simulink model "DK_FlatnessBased_Template0x2810x293"  (R2024a)
settings: Solver=ode3  StartTime=0.0  StopTime=inf  FixedStep=1e-3  RelTol=1e-5  EnableMultiTasking=on
PostLoadFcn:
  | , if any(exist('dsrtsu_mdlpostloadfcn', 'file') == [2, 3, 6]), try dsrtsu_mdlpostloadfcn('Execute', bdroot); catch fprintf('Error in PostLoadFcn (dsrtsu_mdlpostloadfcn) for model "%s":\n %s\n', bdroot, lasterr); end, end,
InitFcn:
  | k3 = -2;
  | k2 = 3;
  | k1 = 0;
  | k0 = 0;
  | 
  | Kp1 = 0.1;
  | Ki1 = 1;
  | Kp2 = 0.01;
  | Ki2 = 0.1;
  | T = 1;
  | delta_t=0.005;
  | 
  | phi_d=.5;
  | phi_0=0;
  | 
  | Phi_LHP = 0;
  | R = 2.0;
  | Cm = 4.19*exp(-3);
  | L = 20*exp(-6);
  | J = 1.7*exp(-6);
  | Cf = 2.2*exp(-4);
  | D = 1*exp(-7);
  | Mfr = 1*exp(-6);
  | Mpre = 1*exp(-6);
  | 
  | %p0=730000;
  | %p1=23300;
  | p0 = 550000;
  | p1 = 21500;
  | p2=260;
  | 
  | % BesselPole Polynom 4. Ordnung
  | bessel_poles_4 = [-0.6573+0.8302i  ,      -0.6573-0.8302i   ,      -0.9047+0.2711i   ,   -0.9047-0.2711i ]
  | a = poly(bessel_poles_4*15);
undefined symbols (not defined in the file): Ki, Kp, phi, ts
libraries: rtilib1104 x4
settings Model: DSRTSU_INTERNAL_RTI_VER=460  DSRTSU_INTERNAL_RTI_TYPE=rti1104  DSRTSU_INTERNAL_RTIFPGA=50  Creator=7eus  LastModifiedBy=danie
settings SolverCC: AlgebraicLoopSolver=TrustRegion
settings DataIOCC: LimitDataPoints=on  SaveFormat=Array  SignalLoggingSaveFormat=ModelDataLogs  ReturnWorkspaceOutputs=off
settings OptimizationCC: BlockReduction=off  OptimizeBlockIOStorage=off  BufferReuse=off  GlobalBufferReuse=off  ExpressionFolding=off  ExpressionDepthLimit=2147483647  LocalBlockOutputs=off  LifeSpan=inf
settings DebuggingCC: AlgebraicLoopMsg=none  UnderspecifiedInitializationDetection=Classic  MergeDetectMultiDrivingBlocksExec=none  FcnCallInpInsideContextMsg=warning  UnconnectedInputMsg=warning  UnconnectedOutputMsg=warning  UnconnectedLineMsg=warning  StateNameClashWarn=warning  SFUnexpectedBacktrackingDiag=warning  SFNoUnconditionalDefaultTransitionDiag=warning  SFExecutionAtInitializationDiag=none  ArithmeticOperatorsInVariantConditions=warning
settings HardwareCC: ProdBitPerPointer=32  ProdBitPerSizeT=32  ProdBitPerPtrDiffT=32  ProdLargestAtomicFloat=None  ProdEndianess=BigEndian  ProdWordSize=32  ProdHWDeviceType=Generic->Custom  TargetIntDivRoundTo=Zero  TargetEndianess=BigEndian  TargetHWDeviceType=Generic->Custom
settings ModelReferenceCC: EnableRefExpFcnMdlSchedulingChecks=on  PropagateSignalLabelsOutOfModel=off
settings SFSimCC: SimUseLocalCustomCode=off  CustomCodeUndefinedFunction=UseInterfaceOnly
settings RTWCC: Description=dSPACE DS1104 Hardware Platform  SystemTargetFile=rti1104.tlc  MakeCommand=make_rti  TemplateMakefile=rti1104.tmf  RTWUseLocalCustomCode=off  GPUComputeCapability=3.5  DLArmComputeVersion=19.05
settings CodeAppCC: StateflowObjectComments=on
settings STFCustomTargetCC: TargetLangStandard=C89/C90 (ANSI)  ParMdlRefBuildCompliant=on  UseToolchainInfoCompliant=off  SystemTargetFile=rti1104.tlc
settings GRTTargetCC: TargetLangStandard=C89/C90 (ANSI)  CompOptLevelCompliant=off  ConcurrentExecutionCompliant=off  CombineOutputUpdateFcns=off  MatFileLogging=off  CPPClassGenCompliant=off  GRTInterface=on  UseToolchainInfoCompliant=off  ExtModeMexFile=noextcomm
settings ConfigComp: CovMetricSettings=dw  CovSaveCumulativeToWorkspaceVar=on  CovSaveSingleToWorkspaceVar=on  CovExternalEMLEnable=off

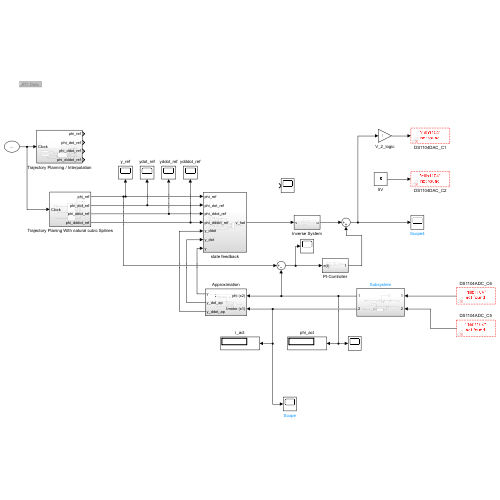
[thumbnail: Simulink's stored preview of the top-level diagram]
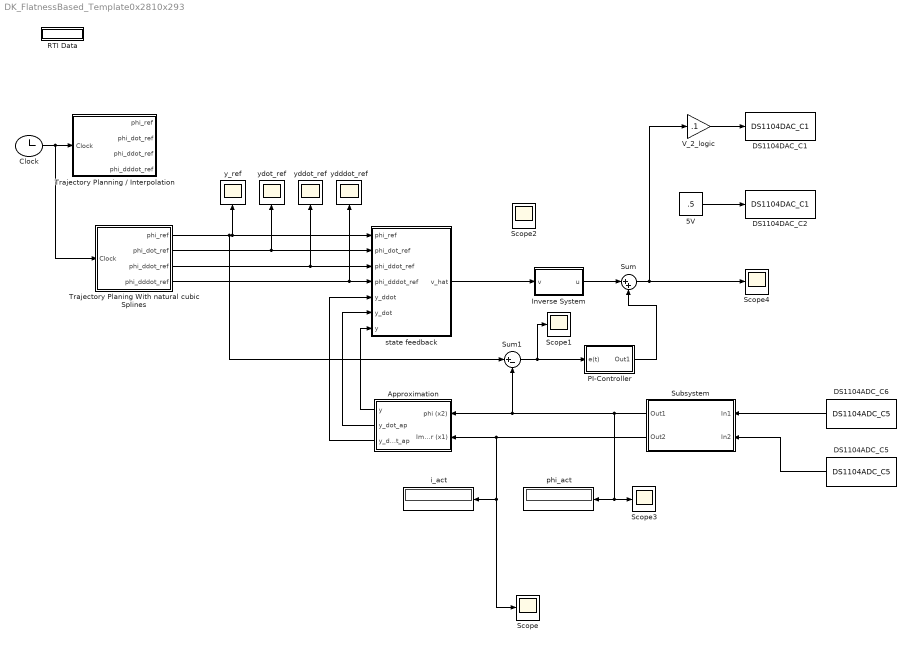
== system DK_FlatnessBased_Template0x2810x293 ==
  5V : Constant  Value=.5
  Approximation : Subsystem
  Clock : Clock
  DS1104ADC_C5 : rtilib1104/DS1104 MASTER PPC/DS1104ADC_C5  ChannelNo=5  TriggerMode=0  Reserved1=[]  Reserved2=[]  Reserved3=[]  Reserved4=[]  DialogFcn=gui1104adc  UnitName={ 'DS1104ADC_C' }  UnitValues={ 5 }  DSProperties=struct('RTI',struct('Version',uint32(1),'BlockType',struct('isSLSource',uint8(1),'isSLSink',uint8(0),'isHWSource',uint8(1),'isHWSink',uint8(0),'isSetup',uint8(0),'isInline',uint8(1),'isNonInline',uint8(0),'isInterrupt',uint8(0),'isChannelwise',uint8(1)),'IOBoardType','DS1104MASTER','UnitType','ADC','Identifier','ADC','DialogType','ML','BlockSet','NONE','SlaveProcessor','NONE'))
  DS1104ADC_C6 : rtilib1104/DS1104 MASTER PPC/DS1104ADC_C5  ChannelNo=6  TriggerMode=0  Reserved1=[]  Reserved2=[]  Reserved3=[]  Reserved4=[]  DialogFcn=gui1104adc  UnitName={ 'DS1104ADC_C' }  UnitValues={6}  DSProperties=struct('RTI',struct('Version',uint32(1),'BlockType',struct('isSLSource',uint8(1),'isSLSink',uint8(0),'isHWSource',uint8(1),'isHWSink',uint8(0),'isSetup',uint8(0),'isInline',uint8(1),'isNonInline',uint8(0),'isInterrupt',uint8(0),'isChannelwise',uint8(1)),'IOBoardType','DS1104MASTER','UnitType','ADC','Identifier','ADC','DialogType','ML','BlockSet','NONE','SlaveProcessor','NONE'))
  DS1104DAC_C1 : rtilib1104/DS1104 MASTER PPC/DS1104DAC_C1  ChannelNo=1  InitValue=0  TermMode=0  TermValue=0  Reserved1=[]  Reserved2=[]  Reserved3=[]  Reserved4=[]  DialogFcn=gui1104dac  UnitName={ 'DS1104DAC_C'}  UnitValues={ 1 }  DSProperties=struct('RTI',struct('Version',uint32(1),'BlockType',struct('isSLSource',uint8(0),'isSLSink',uint8(1),'isHWSource',uint8(0),'isHWSink',uint8(1),'isSetup',uint8(0),'isInline',uint8(1),'isNonInline',uint8(0),'isInterrupt',uint8(0),'isChannelwise',uint8(1)),'IOBoardType','DS1104MASTER','UnitType','DAC','Identifier','DAC','DialogType','ML','BlockSet','NONE','SlaveProcessor','NONE'))
  DS1104DAC_C2 : rtilib1104/DS1104 MASTER PPC/DS1104DAC_C1  ChannelNo=2  InitValue=0  TermMode=0  TermValue=0  Reserved1=[]  Reserved2=[]  Reserved3=[]  Reserved4=[]  DialogFcn=gui1104dac  UnitName={ 'DS1104DAC_C'}  UnitValues={2}  DSProperties=struct('RTI',struct('Version',uint32(1),'BlockType',struct('isSLSource',uint8(0),'isSLSink',uint8(1),'isHWSource',uint8(0),'isHWSink',uint8(1),'isSetup',uint8(0),'isInline',uint8(1),'isNonInline',uint8(0),'isInterrupt',uint8(0),'isChannelwise',uint8(1)),'IOBoardType','DS1104MASTER','UnitType','DAC','Identifier','DAC','DialogType','ML','BlockSet','NONE','SlaveProcessor','NONE'))
  Inverse System : Subsystem
  PI-Controller : Subsystem
  RTI Data : Subsystem  Tag=struct('RTIDataServer',struct('RTIDataServerVs','2','RTIModelDescription','struct(''main'',''DK_FlatnessBased_Template'',''sub'',''DK_FlatnessBased_Template'',''isMp'',0)'))  LoadFcn="if exist('rtidc'), try,  rtidc('DataHostBlockClbLoad', gcbh); catch, disp(['Warning: ''LoadFcn'' for RTI Data block failed: ' lasterr]); end, end,"  mask(RTI_DATA_HOST){}
      mask help:
      | RTI Data Block.
      | This block is used by RTI to store internal model-dependent data.
      | Please keep this block on the root level of the model. Deleting this block will result in data loss.
      |
      | NEVER DELETE OR COPY THIS BLOCK!
      settings: CopyFcn="if exist('rtidc'), try,  rtidc('DataHostBlockClbCopy', gcbh); catch, disp(['Warning: ''CopyFcn'' for RTI Data block failed: ' lasterr]); end, end,"  DeleteFcn="if exist('rtidc'), try,  rtidc('DataHostBlockClbDelete', gcbh); catch, disp(['Warning: ''DeleteFcn'' for RTI Data block failed: ' lasterr]); end, end,"  ModelCloseFcn="if exist('rtidc'), try,  rtidc('DataHostBlockClbModelClose', gcbh); catch, disp(['Warning: ''ModelCloseFcn'' for RTI Data block failed: ' lasterr]); end, end,"  PreSaveFcn="if exist('rtidc'), try,  rtidc('DataHostBlockClbPreSave', gcbh); catch, disp(['Warning: ''PreSaveFcn'' for RTI Data block failed: ' lasterr]); end, end,"  PostSaveFcn="if exist('rtidc'), try,  rtidc('DataHostBlockClbPostSave', gcbh); catch, disp(['Warning: ''PostSaveFcn'' for RTI Data block failed: ' lasterr]); end, end,"  NameChangeFcn="if exist('rtidc'), try,  rtidc('DataHostBlockClbNameChange', gcbh); catch, disp(['Warning: ''NameChangeFcn'' for RTI Data block failed: ' lasterr]); end, end,"
      mask Help:
      | RTI Data Block.
      | This block is used by RTI to store internal model-dependent data.
      | Please keep this block on the root level of the model. Deleting this block will result in data loss.
      | 
      | NEVER DELETE OR COPY THIS BLOCK!
      mask Display: text(0.5, 0.5, 'RTI Data', 'HorizontalAlignment', 'center');
  Scope{,1..4} (5 alike) : Scope
  Subsystem : Subsystem
  Sum : Sum  Inputs=|++
  Sum1 : Sum  Inputs=|+-
  Trajectory Planing With natural cubic Splines : Subsystem
  Trajectory Planning / Interpolation : Subsystem
  V_2_logic : Gain  Gain=.1
  i_act : Display
  phi_act : Display
  state feedback : Subsystem
  y_ref : Scope
  ydddot_ref : Scope
  yddot_ref : Scope
  ydot_ref : Scope
  wires:
  5V/1 -> DS1104DAC_C2/1
  V_2_logic/1 -> DS1104DAC_C1/1
  Trajectory Planing With natural cubic Splines/1(phi_ref) -> y_ref/1, state feedback/1(phi_ref), Sum1/1
  Trajectory Planing With natural cubic Splines/4(phi_dddot_ref) -> ydddot_ref/1, state feedback/4(phi_dddot_ref)
  Approximation/3(y_ddot_ap) -> state feedback/5(y_ddot)
  Approximation/2(y_dot_ap) -> state feedback/6(y_dot)
  Clock/1 -> Trajectory Planing With natural cubic Splines/1(Clock), Trajectory Planning / Interpolation/1(Clock)
  Trajectory Planing With natural cubic Splines/2(phi_dot_ref) -> ydot_ref/1, state feedback/2(phi_dot_ref)
  Approximation/1(y) -> state feedback/7(y)
  Trajectory Planing With natural cubic Splines/3(phi_ddot_ref) -> yddot_ref/1, state feedback/3(phi_ddot_ref)
  state feedback/1(v_hat) -> Inverse System/1(v)
  PI-Controller/1(Out1) -> Sum/2
  Inverse System/1(u) -> Sum/1
  Sum/1 -> Scope4/1, V_2_logic/1
  Sum1/1 -> PI-Controller/1(e(t)), Scope1/1
  Subsystem/1(Out1) -> Sum1/2, Approximation/1(phi (x2)), Scope3/1, phi_act/1
  Subsystem/2(Out2) -> Scope/1, i_act/1, Approximation/2(Imotor (x1))
  DS1104ADC_C6/1 -> Subsystem/1(In1)
  DS1104ADC_C5/1 -> Subsystem/2(In2)

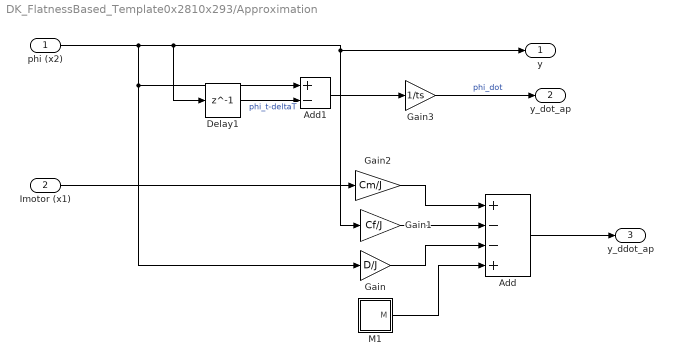
== system DK_FlatnessBased_Template0x2810x293/Approximation ==
  phi (x2) : Inport
  Imotor (x1) : Inport  Port=2
  Add : Sum  Inputs=+--+
  Add1 : Sum  Inputs=+-
  Delay1 : Delay  DelayLength=1  SampleTime=ts
  Gain : Gain  Gain=D/J
  Gain1 : Gain  Gain=Cf/J
  Gain2 : Gain  Gain=Cm/J
  Gain3 : Gain  Gain=1/ts
  M1 : Subsystem
  y : Outport
  y_dot_ap : Outport  Port=2
  y_ddot_ap : Outport  Port=3
  wires:
  phi (x2)/1 -> Gain/1, Add1/1, Delay1/1, Gain1/1, y/1
  M1/1(M) -> Add/4
  Gain/1 -> Add/3
  Gain1/1 -> Add/2
  Gain2/1 -> Add/1
  Imotor (x1)/1 -> Gain2/1
  Add/1 -> y_ddot_ap/1
  Gain3/1 -> y_dot_ap/1  "phi_dot"
  Add1/1 -> Gain3/1
  Delay1/1 -> Add1/2  "phi_t-deltaT"

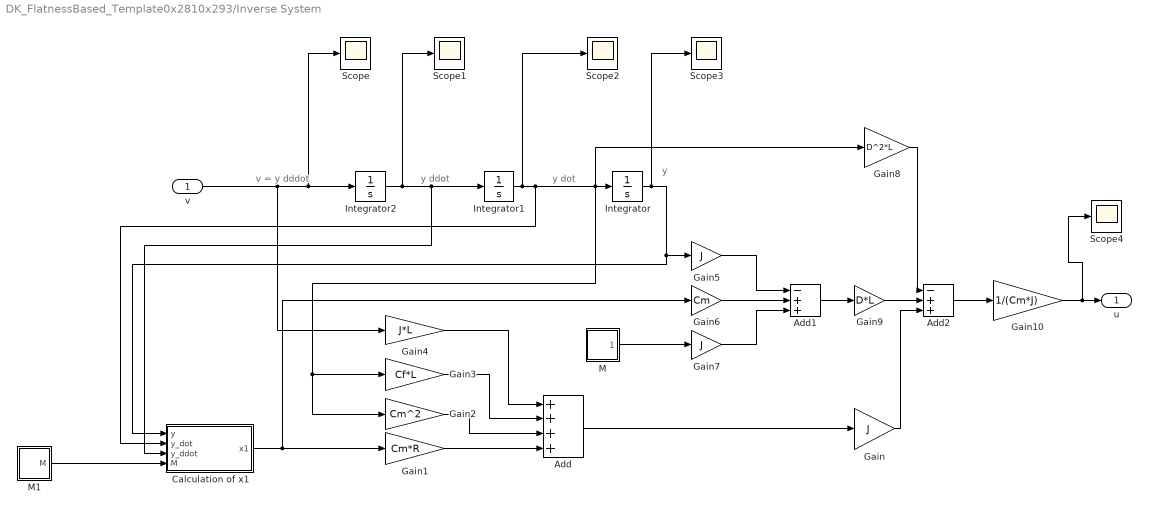
== system DK_FlatnessBased_Template0x2810x293/Inverse System ==
  note: v = y dddot
  note: y ddot
  note: y dot
  note: y
  v : Inport
  Add : Sum  Inputs=++++
  Add1 : Sum  Inputs=-++
  Add2 : Sum  Inputs=-++
  Calculation of x1 : Subsystem
  Gain : Gain  Gain=J
  Gain1 : Gain  Gain=Cm*R
  Gain10 : Gain  Gain=1/(Cm*J)
  Gain2 : Gain  Gain=Cm^2
  Gain3 : Gain  Gain=Cf*L
  Gain4 : Gain  Gain=J*L
  Gain5 : Gain  Gain=J
  Gain6 : Gain  Gain=Cm
  Gain7 : Gain  Gain=J
  Gain8 : Gain  Gain=D^2*L
  Gain9 : Gain  Gain=D*L
  Integrator : Integrator
  Integrator1 : Integrator
  Integrator2 : Integrator
  M : Subsystem
  M1 : Subsystem
  Scope{,1..4} (5 alike) : Scope
  u : Outport
  wires:
  Integrator1/1 -> Scope2/1, Calculation of x1/2(y_dot), Gain8/1, Gain2/1, Gain3/1, Integrator/1
  Integrator2/1 -> Scope1/1, Calculation of x1/3(y_ddot), Integrator1/1
  Integrator/1 -> Scope3/1, Calculation of x1/1(y), Gain5/1
  v/1 -> Scope/1, Integrator2/1, Gain4/1
  Add/1 -> Gain/1
  Gain1/1 -> Add/4
  Gain2/1 -> Add/3
  Gain3/1 -> Add/2
  Gain4/1 -> Add/1
  M/1(Out1) -> Gain7/1
  Gain7/1 -> Add1/3
  Gain6/1 -> Add1/2
  Gain5/1 -> Add1/1
  Add1/1 -> Gain9/1
  Gain10/1 -> Scope4/1, u/1
  Add2/1 -> Gain10/1
  Gain/1 -> Add2/3
  Gain9/1 -> Add2/2
  Gain8/1 -> Add2/1
  Calculation of x1/1(x1) -> Gain6/1, Gain1/1
  M1/1(M) -> Calculation of x1/4(M)

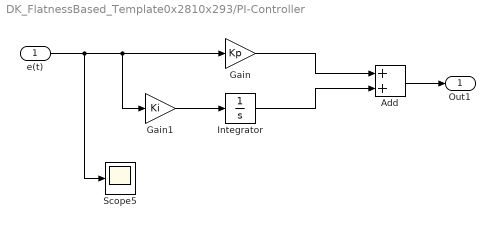
== system DK_FlatnessBased_Template0x2810x293/PI-Controller ==
  e(t) : Inport
  Add : Sum
  Gain : Gain  Gain=Kp
  Gain1 : Gain  Gain=Ki
  Integrator : Integrator
  Scope5 : Scope
  Out1 : Outport
  wires:
  Add/1 -> Out1/1
  e(t)/1 -> Scope5/1, Gain1/1, Gain/1
  Gain/1 -> Add/1
  Integrator/1 -> Add/2
  Gain1/1 -> Integrator/1

== system DK_FlatnessBased_Template0x2810x293/RTI Data ==
  RTI Data Store : Subsystem  mask(RTI_DATA_STORE){}
      mask help:
      | RTI Data Store Block. This block is used by RTI to store internal model dependent data. Deleting this block will result in data loss.
      |
      | NEVER DELETE, COPY, OR MODIFY THIS BLOCK!
      mask Help:
      | RTI Data Store Block. This block is used by RTI to store internal model dependent data. Deleting this block will result in data loss.
      | 
      | NEVER DELETE, COPY, OR MODIFY THIS BLOCK!
      mask Display: text(0.5, 0.5, ' ', 'HorizontalAlignment', 'center');

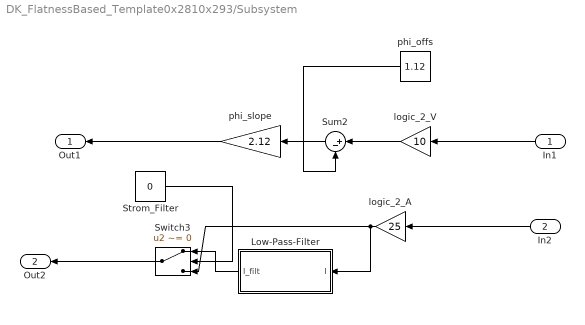
== system DK_FlatnessBased_Template0x2810x293/Subsystem ==
  In1 : Inport
  In2 : Inport  Port=2
  Low-Pass-Filter : Subsystem
  Strom_Filter : Constant  Value=0
  Sum2 : Sum  Inputs=|+-
  Switch3 : Switch  Criteria=u2 ~= 0  SaturateOnIntegerOverflow=off  InputSameDT=off
  logic_2_A : Gain  Gain=25
  logic_2_V : Gain  Gain=10
  phi_offs : Constant  Value=1.12
  phi_slope : Gain  Gain=2.12
  Out1 : Outport
  Out2 : Outport  Port=2
  wires:
  phi_slope/1 -> Out1/1
  Switch3/1 -> Out2/1
  phi_offs/1 -> Sum2/2
  Low-Pass-Filter/1(I_filt) -> Switch3/1
  logic_2_A/1 -> Switch3/3, Low-Pass-Filter/1(I)
  In1/1 -> logic_2_V/1
  Sum2/1 -> phi_slope/1
  logic_2_V/1 -> Sum2/1
  Strom_Filter/1 -> Switch3/2
  In2/1 -> logic_2_A/1

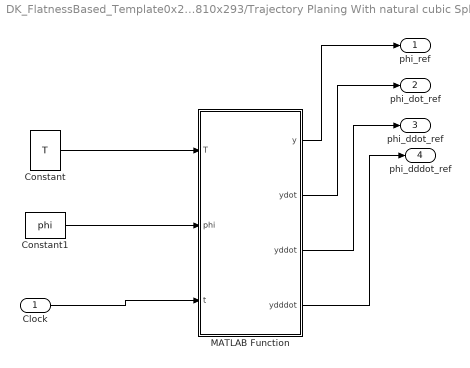
== system DK_FlatnessBased_Template0x2810x293/Trajectory Planing With natural cubic Splines ==
  Clock : Inport
  Constant : Constant  Value=T
  Constant1 : Constant  Value=phi
  MATLAB Function : MATLAB Function  TreatAsAtomicUnit=on
  phi_ref : Outport
  phi_dot_ref : Outport  Port=2
  phi_ddot_ref : Outport  Port=3
  phi_dddot_ref : Outport  Port=4
  wires:
  MATLAB Function/4(ydddot) -> phi_dddot_ref/1
  MATLAB Function/2(ydot) -> phi_dot_ref/1
  MATLAB Function/1(y) -> phi_ref/1
  MATLAB Function/3(yddot) -> phi_ddot_ref/1
  Clock/1 -> MATLAB Function/3(t)
  Constant1/1 -> MATLAB Function/2(phi)
  Constant/1 -> MATLAB Function/1(T)

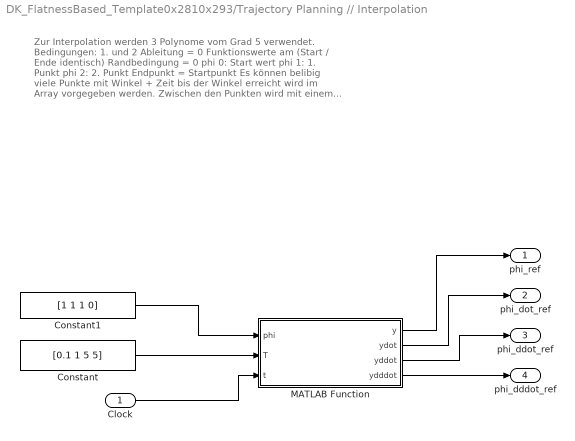
== system DK_FlatnessBased_Template0x2810x293/Trajectory Planning // Interpolation ==
  note: Zur Interpolation werden 3 Polynome vom Grad 5 verwendet.
      |
      | Bedingungen: 1. und 2 Ableitung = 0
      | 			 Funktionswerte am (Start / Ende identisch)
      | 			 Randbedingung = 0
      |
      | phi 0: Start wert
      | phi 1: 1. Punkt
      | phi 2: 2. Punkt
      | Endpunkt = Startpunkt
      |
      | Es können belibig viele Punkte mit Winkel + Zeit bis der Winkel erreicht wird im Array vorgegeben werden.
      |
      | Zwischen den Punkten wird mit einem Polynom 5. Ordnung interpoliert
  Clock : Inport
  Constant : Constant  Value=[0.1 1 5 5]  VectorParams1D=off
  Constant1 : Constant  Value=[1 1 1 0]
  MATLAB Function : MATLAB Function  TreatAsAtomicUnit=on
  phi_ref : Outport
  phi_dot_ref : Outport  Port=2
  phi_ddot_ref : Outport  Port=3
  phi_dddot_ref : Outport  Port=4
  wires:
  MATLAB Function/1(y) -> phi_ref/1
  MATLAB Function/2(ydot) -> phi_dot_ref/1
  MATLAB Function/3(yddot) -> phi_ddot_ref/1
  MATLAB Function/4(ydddot) -> phi_dddot_ref/1
  Clock/1 -> MATLAB Function/3(t)
  Constant/1 -> MATLAB Function/2(T)
  Constant1/1 -> MATLAB Function/1(phi)

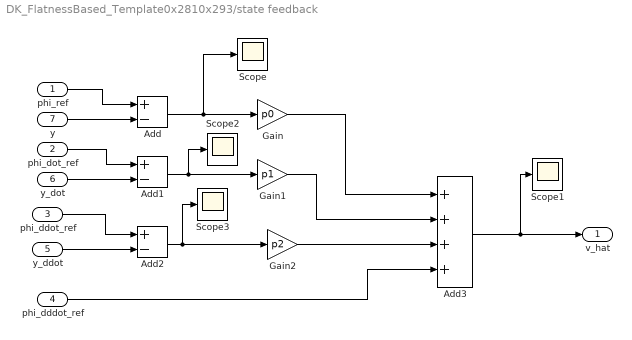
== system DK_FlatnessBased_Template0x2810x293/state feedback ==
  phi_ref : Inport
  phi_dot_ref : Inport  Port=2
  phi_ddot_ref : Inport  Port=3
  phi_dddot_ref : Inport  Port=4
  y_ddot : Inport  Port=5
  y_dot : Inport  Port=6
  y : Inport  Port=7
  Add : Sum  Inputs=+-
  Add1 : Sum  Inputs=+-
  Add2 : Sum  Inputs=+-
  Add3 : Sum  Inputs=++++
  Gain : Gain  Gain=p0
  Gain1 : Gain  Gain=p1
  Gain2 : Gain  Gain=p2
  Scope{,1..3} (4 alike) : Scope
  v_hat : Outport
  wires:
  Add1/1 -> Scope2/1, Gain1/1
  Add/1 -> Scope/1, Gain/1
  Add2/1 -> Scope3/1, Gain2/1
  Gain/1 -> Add3/1
  Gain1/1 -> Add3/2
  Gain2/1 -> Add3/3
  phi_dddot_ref/1 -> Add3/4
  Add3/1 -> Scope1/1, v_hat/1
  y/1 -> Add/2
  phi_ref/1 -> Add/1
  phi_dot_ref/1 -> Add1/1
  y_dot/1 -> Add1/2
  y_ddot/1 -> Add2/2
  phi_ddot_ref/1 -> Add2/1

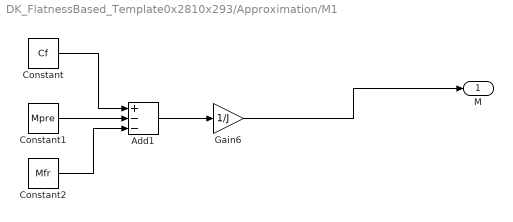
== system DK_FlatnessBased_Template0x2810x293/Approximation/M1 ==
  Add1 : Sum  Inputs=+--
  Constant : Constant  Value=Cf
  Constant1 : Constant  Value=Mpre
  Constant2 : Constant  Value=Mfr
  Gain6 : Gain  Gain=1/J
  M : Outport
  wires:
  Constant/1 -> Add1/1
  Add1/1 -> Gain6/1
  Constant2/1 -> Add1/3
  Constant1/1 -> Add1/2
  Gain6/1 -> M/1

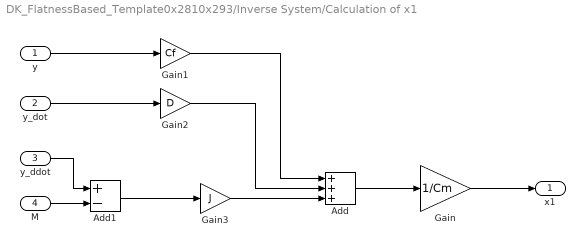
== system DK_FlatnessBased_Template0x2810x293/Inverse System/Calculation of x1 ==
  y : Inport
  y_dot : Inport  Port=2
  y_ddot : Inport  Port=3
  M : Inport  Port=4
  Add : Sum  Inputs=+++
  Add1 : Sum  Inputs=+-
  Gain : Gain  Gain=1/Cm
  Gain1 : Gain  Gain=Cf
  Gain2 : Gain  Gain=D
  Gain3 : Gain  Gain=J
  x1 : Outport
  wires:
  Add/1 -> Gain/1
  Gain/1 -> x1/1
  y/1 -> Gain1/1
  Gain1/1 -> Add/1
  y_dot/1 -> Gain2/1
  Gain2/1 -> Add/2
  y_ddot/1 -> Add1/1
  Add1/1 -> Gain3/1
  Gain3/1 -> Add/3
  M/1 -> Add1/2

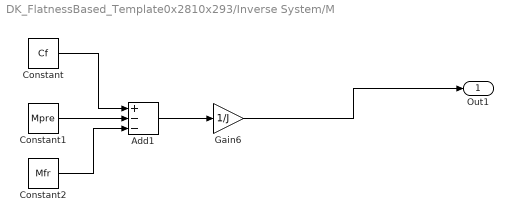
== system DK_FlatnessBased_Template0x2810x293/Inverse System/M ==
  Add1 : Sum  Inputs=+--
  Constant : Constant  Value=Cf
  Constant1 : Constant  Value=Mpre
  Constant2 : Constant  Value=Mfr
  Gain6 : Gain  Gain=1/J
  Out1 : Outport
  wires:
  Constant/1 -> Add1/1
  Add1/1 -> Gain6/1
  Constant2/1 -> Add1/3
  Constant1/1 -> Add1/2
  Gain6/1 -> Out1/1

== system DK_FlatnessBased_Template0x2810x293/Inverse System/M1 ==
  Add1 : Sum  Inputs=+--
  Constant : Constant  Value=Cf
  Constant1 : Constant  Value=Mpre
  Constant2 : Constant  Value=Mfr
  Gain6 : Gain  Gain=1/J
  M : Outport
  wires:
  Constant/1 -> Add1/1
  Add1/1 -> Gain6/1
  Constant2/1 -> Add1/3
  Constant1/1 -> Add1/2
  Gain6/1 -> M/1

== system DK_FlatnessBased_Template0x2810x293/RTI Data/RTI Data Store ==
  RTI Data Store : Subsystem  mask(RTI_DATA_STORE){}
      mask help:
      | RTI Data Store Block. This block is used by RTI to store internal model dependent data. Deleting this block will result in data loss.
      |
      | NEVER DELETE, COPY, OR MODIFY THIS BLOCK!
      mask Help:
      | RTI Data Store Block. This block is used by RTI to store internal model dependent data. Deleting this block will result in data loss.
      | 
      | NEVER DELETE, COPY, OR MODIFY THIS BLOCK!
      mask Display: text(0.5, 0.5, ' ', 'HorizontalAlignment', 'center');

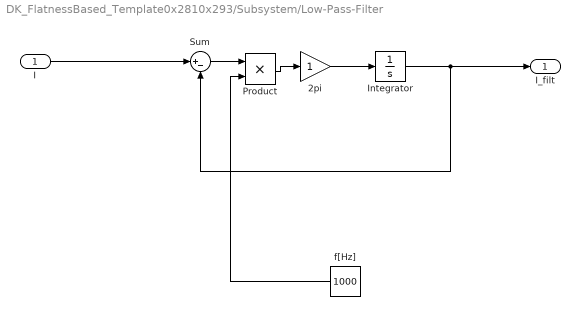
== system DK_FlatnessBased_Template0x2810x293/Subsystem/Low-Pass-Filter ==
  I : Inport
  2pi : Gain
  Integrator : Integrator
  Product : Product  RndMeth=Zero
  Sum : Sum  Inputs=|+-
  f[Hz] : Constant  Value=1000
  I_filt : Outport
  wires:
  Integrator/1 -> I_filt/1, Sum/2
  I/1 -> Sum/1
  2pi/1 -> Integrator/1
  Sum/1 -> Product/1
  Product/1 -> 2pi/1
  f[Hz]/1 -> Product/2

== system DK_FlatnessBased_Template0x2810x293/RTI Data/RTI Data Store/RTI Data Store ==
  RTI Data Store : Subsystem  mask(RTI_DATA_STORE){}
      mask help:
      | RTI Data Store Block. This block is used by RTI to store internal model dependent data. Deleting this block will result in data loss.
      |
      | NEVER DELETE, COPY, OR MODIFY THIS BLOCK!
      mask Help:
      | RTI Data Store Block. This block is used by RTI to store internal model dependent data. Deleting this block will result in data loss.
      | 
      | NEVER DELETE, COPY, OR MODIFY THIS BLOCK!
      mask Display: text(0.5, 0.5, ' ', 'HorizontalAlignment', 'center');

== system DK_FlatnessBased_Template0x2810x293/RTI Data/RTI Data Store/RTI Data Store/RTI Data Store ==
  RTI Data Store : Subsystem  mask(RTI_DATA_STORE){}
      mask help:
      | RTI Data Store Block. This block is used by RTI to store internal model dependent data. Deleting this block will result in data loss.
      |
      | NEVER DELETE, COPY, OR MODIFY THIS BLOCK!
      mask Help:
      | RTI Data Store Block. This block is used by RTI to store internal model dependent data. Deleting this block will result in data loss.
      | 
      | NEVER DELETE, COPY, OR MODIFY THIS BLOCK!
      mask Display: text(0.5, 0.5, ' ', 'HorizontalAlignment', 'center');

== system DK_FlatnessBased_Template0x2810x293/RTI Data/RTI Data Store/RTI Data Store/RTI Data Store/RTI Data Store ==

== matlab function DK_FlatnessBased_Template0x2810x293/Trajectory Planning // Interpolation/MATLAB Function ==
  data: phi input; y output; T input; t input; ydot output; yddot output; ydddot output
function [y, ydot, yddot, ydddot] = fcn(phi, T, t)
   
    % Gesamtzeit aller Intervalle
    total_duration = sum(T);
    
    % Modulo-Operation, um t zyklisch zu machen
    t_mod = mod(t, total_duration);

    t_start = 0; % Init start time
    
    % Durchlaufe alle Intervalle
    for i = 1:length(T)
        % Bestimme das aktuelle Intervall
        t_end = t_start + T(i);
        
        % Prüfe, ob t_mod in das aktuelle Intervall fällt
        if t_mod < t_end
            % Evaluiere das entsprechende Polynom
            if i <= 1
                coeffs = compute_coeffs(0, phi(i), T(i));
            else
                coeffs = compute_coeffs(phi(i-1), phi(i), T(i));
            end    
            % Berechnung der Koeffizienten der Ableitungen
            coeffs_first_derivative  = polyder(coeffs);
            coeffs_second_derivative = polyder(coeffs_first_derivative); 
            coeffs_third_derivative  = polyder(coeffs_second_derivative); % dritte Ableitung
            % Auswertung zum Zeitpunkt t (eval_time)
            y      = polyval(coeffs, t_mod - t_start);
            ydot   = polyval(coeffs_first_derivative, t_mod - t_start);
            yddot  = polyval(coeffs_second_derivative, t_mod - t_start);
            ydddot = polyval(coeffs_third_derivative, t_mod - t_start);
            return;
        end
        
        % Aktualisiere den Startzeitpunkt für das nächste Intervall
        t_start = t_end;
    end

    % FEHLER FALL
    y      = 0;
    ydot   = 0;
    yddot  = 0;
    ydddot = 0;
    

end

function coeffs = compute_coeffs(phi_0, phi_d, T)
    % Matrix A
    A = [0 0 0 0 0 1;
         T^5 T^4 T^3 T^2 T 1;
         0 0 0 2 0 0;
         0 0 0 0 1 0;
         5*T^4 4*T^3 3*T^2 2*T 1 0;
         20*T^3 12*T^2 2*T 1 0 0];
    
    % Vector b
    b = transpose([phi_0 phi_d 0 0 0 0]);

    % Berechnung der Koeffizienten
    coeffs = A\b;
end

== matlab function DK_FlatnessBased_Template0x2810x293/Trajectory Planing With natural cubic Splines/MATLAB Function ==
  data: T input; phi input; t input; y output; ydot output; yddot output; ydddot output
function [y, ydot, yddot, ydddot] = fcn(T, phi, t)
    
    t_mod = mod(t, max(T));
    % Erstellen der spline-Struktur
    pp = spline(T, phi);

    pp_coder = create_compatible_pp(pp);
    
    % Bestimmen des Funktionswertes zum Zeitpunkt t (bzw. t_mod)
    y = ppval(pp_coder, t_mod);

    % 1. Ableitung 
    d_pp = compute_derivative_pp(pp);
    ydot = ppval(d_pp, t_mod);
    % 2. Ableitung (zweite Ableitung)
    d2_pp = compute_derivative_pp(d_pp);
    yddot = ppval(d2_pp,t_mod);

    % 3. Ableitung (dritte Ableitung)
    d3_pp = compute_derivative_pp(d2_pp);
    ydddot = ppval(d3_pp,t_mod);
end

% ppval ist nicht kompatibel mit dem Simulink coder
% mkpp ermöglicht die Erstellung einer coder kompatiblen verison
function pp_coder = create_compatible_pp(pp)
    % Extract coefficients using unmkpp
    [breaks, coefs, ~, ~, ~] = unmkpp(pp);

    % Create a MATLAB Coder compatible pp form using mkpp
    pp_coder = mkpp(breaks, coefs);
end

function d_pp = compute_derivative_pp(pp)
    [breaks, coefs, l, k, d] = unmkpp(pp);

    % Initialize an empty array to store derivative coefficients
    d_coefs = zeros(size(coefs));

    % Calculate coefficients for the derivative spline
    for i = 1:size(coefs, 2) % Iterate over each polynomial piece
        d_coefs(:, i) = coefs(:, i) * (k-i); % Multiply by the derivative factor
    end

    % Create the derivative spline d_pp
    d_pp = mkpp(breaks, d_coefs);


end
